simulink subsystem "USV_Model"  (R2022a)
settings: Solver=VariableStepAuto  StartTime=0.0  StopTime=10.0  RelTol=1e-3
model mask{x=0, y=0, psi=0}
values from neighbouring files (symbols this model uses):
  y = x1+a0    [ADRC_TD.m]
settings Model: Creator=45489  LastModifiedBy=45489
settings SolverCC: AlgebraicLoopSolver=TrustRegion
settings DebuggingCC: UnconnectedInputMsg=warning  UnconnectedOutputMsg=warning  UnconnectedLineMsg=warning  SFMachineParentedDataDiag=warning

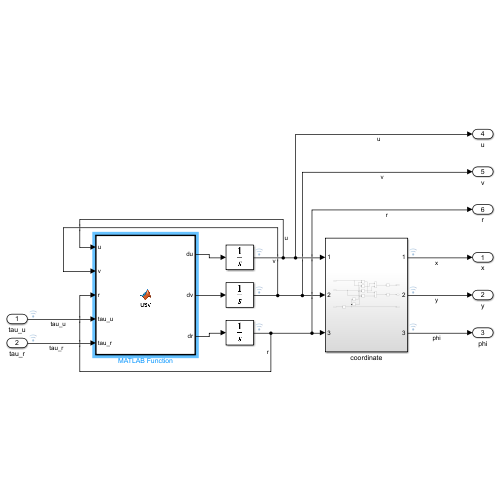
[thumbnail: Simulink's stored preview of the top-level diagram]
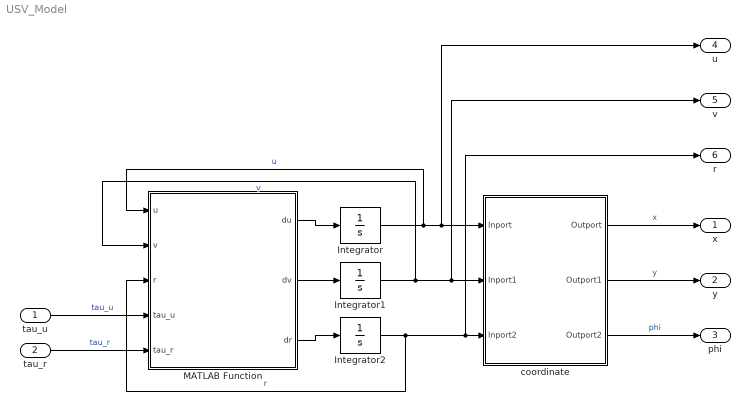
== system USV_Model ==
  tau_u : Inport
  tau_r : Inport  Port=2
  Integrator : Integrator
  Integrator1 : Integrator
  Integrator2 : Integrator
  MATLAB Function : MATLAB Function  TreatAsAtomicUnit=on
  coordinate : Subsystem
  x : Outport
  y : Outport  Port=2
  phi : Outport  Port=3
  u : Outport  Port=4
  v : Outport  Port=5
  r : Outport  Port=6
  wires:
  Integrator/1 -> coordinate/1(Inport), u/1, MATLAB Function/1(u)  "u"
  Integrator1/1 -> coordinate/2(Inport1), v/1, MATLAB Function/2(v)  "v"
  Integrator2/1 -> coordinate/3(Inport2), r/1, MATLAB Function/3(r)  "r"
  MATLAB Function/2(dv) -> Integrator1/1
  coordinate/1(Outport) -> x/1  "x"
  coordinate/3(Outport2) -> phi/1  "phi"
  coordinate/2(Outport1) -> y/1  "y"
  MATLAB Function/3(dr) -> Integrator2/1
  MATLAB Function/1(du) -> Integrator/1
  tau_r/1 -> MATLAB Function/5(tau_r)  "tau_r"
  tau_u/1 -> MATLAB Function/4(tau_u)  "tau_u"

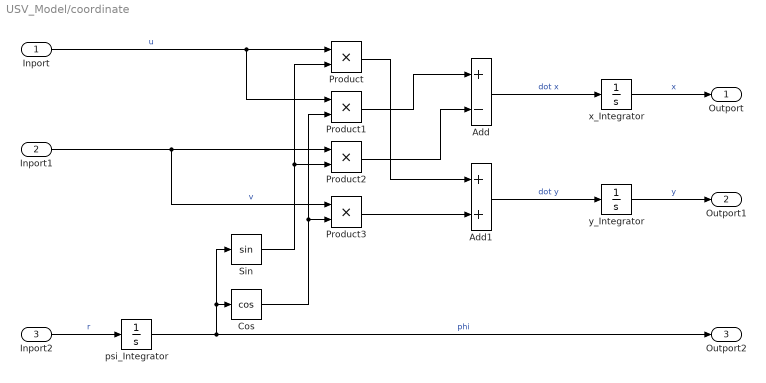
== system USV_Model/coordinate ==
  Inport : Inport
  Inport1 : Inport  Port=2
  Inport2 : Inport  Port=3
  Add : Sum  Inputs=+-
  Add1 : Sum
  Cos : Trigonometry  Operator=cos
  Product{,1..3} (4 alike) : Product
  Sin : Trigonometry
  psi_Integrator : Integrator  InitialCondition=psi
  x_Integrator : Integrator  InitialCondition=x
  y_Integrator : Integrator  InitialCondition=y
  Outport : Outport
  Outport1 : Outport  Port=2
  Outport2 : Outport  Port=3
  wires:
  y_Integrator/1 -> Outport1/1  "y"
  Product/1 -> Add1/1
  Product1/1 -> Add/1
  Inport1/1 -> Product2/1, Product3/1  "v"
  Inport2/1 -> psi_Integrator/1  "r"
  Product3/1 -> Add1/2
  Inport/1 -> Product/1, Product1/1  "u"
  Cos/1 -> Product3/2, Product1/2
  Sin/1 -> Product2/2, Product/2
  Add1/1 -> y_Integrator/1  "dot y"
  Product2/1 -> Add/2
  psi_Integrator/1 -> Outport2/1, Cos/1, Sin/1  "phi"
  Add/1 -> x_Integrator/1  "dot x"
  x_Integrator/1 -> Outport/1  "x"

== matlab function USV_Model/MATLAB Function ==
  data: u input; du output; v input; r input; tau_u input; tau_r input; dv output; dr output
function [du, dv, dr] = usv(u, v, r, tau_u, tau_r)
    du=0.1*r^2+v*r+tau_u/33-5*u/33;
    dv=50/967*r-10/967*tau_r-5000/31911*v-r*u;
    dr=100/967*tau_r-500/967*r+50/967*v;
